simulink model "modulacao_delta"  (Simulink 7.7)
settings: Solver=FixedStepDiscrete  StartTime=0  StopTime=2  RelTol=1e-3
libraries: simulink x2, dspsigops x1
settings Model: Creator=Cliente  LastModifiedBy=Cliente

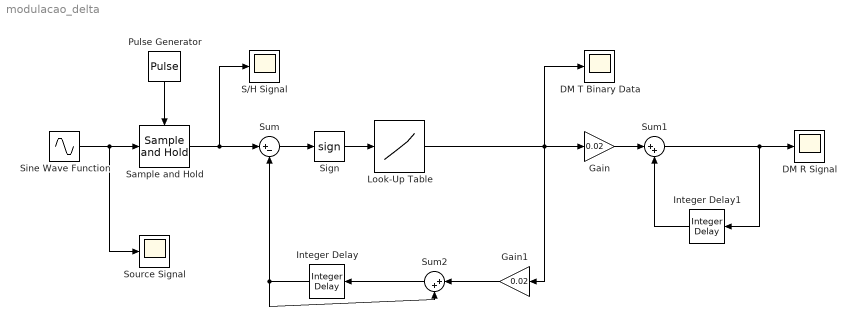
== system modulacao_delta ==
  DM R Signal : Scope
      settings: SaveName=ScopeData3
  DM T Binary Data : Scope
      settings: SaveName=ScopeData2
  Gain : Gain  Gain=0.02
  Gain1 : Gain  Gain=0.02
  Integer Delay : simulink/Discrete/Integer Delay  NumDelays=5  InputProcessing=Inherited  vinit=0.0  samptime=-1
  Integer Delay1 : simulink/Discrete/Integer Delay  NumDelays=5  InputProcessing=Inherited  vinit=0.0  samptime=-1
  Look-Up Table : Lookup  InputValues=[-1;0;1]  Table=[-1,-1,1]  SaturateOnIntegerOverflow=on
  Pulse Generator : DiscretePulseGenerator  PulseType=Time based  Period=5e-4  PulseWidth=20
  S/H Signal : Scope
  Sample and Hold : dspsigops/Sample and Hold  SystemSampleTime=-1  trig=Rising edge  initCond=0  latchinput=off
  Sign : Signum
  Sine Wave Function : Sin  Frequency=4*pi  SampleTime=1e-4
  Source Signal : Scope
  Sum : Sum  Inputs=|+-
  Sum1 : Sum  Inputs=|++
  Sum2 : Sum  Inputs=|++
  wires:
  Sine Wave Function/1 -> Sample and Hold/1, Source Signal/1
  Pulse Generator/1 -> Sample and Hold/Trigger
  Sample and Hold/1 -> Sum/1, S/H Signal/1
  Sum/1 -> Sign/1
  Sign/1 -> Look-Up Table/1
  Look-Up Table/1 -> Gain/1, Gain1/1, DM T Binary Data/1
  Gain/1 -> Sum1/1
  Sum1/1 -> Integer Delay1/1, DM R Signal/1
  Gain1/1 -> Sum2/1
  Sum2/1 -> Integer Delay/1
  Integer Delay/1 -> Sum2/2, Sum/2
  Integer Delay1/1 -> Sum1/2
